simulink model "emerg_imp"  (R2018a)
settings: Solver=FixedStepDiscrete  StartTime=0.0  StopTime=10.0  RelTol=1e-3
settings Model: Creator=BEAR  LastModifiedBy=BEAR
settings OptimizationCC: DefaultParameterBehavior=Inlined  UseDivisionForNetSlopeComputation=on  UseFloatMulNetSlope=on  InlineInvariantSignals=on  PassReuseOutputArgsAs=Individual arguments  ZeroExternalMemoryAtStartup=off  ZeroInternalMemoryAtStartup=off  NoFixptDivByZeroProtection=on  EfficientFloat2IntCast=on  LifeSpan=1  OptimizeBlockOrder=speed  DifferentSizesBufferReuse=on
settings DebuggingCC: ParameterTunabilityLossMsg=error
settings HardwareCC: ProdBitPerLong=64  ProdLongLongMode=on  ProdHWDeviceType=Intel->x86-64 (Mac OS X)
settings SFSimCC: MATLABDynamicMemAlloc=off
settings RTWCC: SystemTargetFile=ert.tlc  TemplateMakefile=ert_default_tmf  GenerateReport=on  IncludeHyperlinkInReport=on  LaunchReport=on  GenerateTraceInfo=on  GenerateTraceReport=on  GenerateTraceReportSl=on  GenerateTraceReportSf=on  GenerateTraceReportEml=on  GenerateCodeMetricsReport=on
settings CodeAppCC: ForceParamTrailComments=on  IgnoreCustomStorageClasses=off  OperatorAnnotations=on  SimulinkDataObjDesc=on  SFDataObjDesc=on  CustomSymbolStrGlobalVar=rt$N$M  CustomSymbolStrType=$N$M  CustomSymbolStrFcn=$N$M$F  CustomSymbolStrMacro=$N$M  InsertBlockDesc=on
settings ERTTargetCC: TargetLangStandard=C99 (ISO)  GenerateSampleERTMain=on  IncludeMdlTerminateFcn=off  CombineSignalStateStructs=on  SupportAbsoluteTime=off  SupportComplex=off  SupportNonInlinedSFcns=on  InlinedParameterPlacement=NonHierarchical  ERTCustomFileTemplate=example_file_process.tlc  ERTFilePackagingFormat=CompactWithDataFile

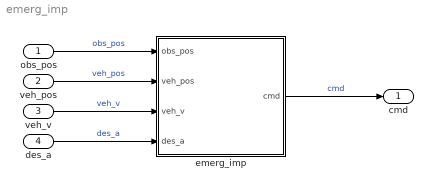
== system emerg_imp ==
  obs_pos : Inport
  veh_pos : Inport  Port=2
  veh_v : Inport  Port=3
  des_a : Inport  Port=4
  emerg_imp : Stateflow chart  TreatAsAtomicUnit=on
  cmd : Outport
  wires:
  obs_pos/1 -> emerg_imp/1(obs_pos)  "obs_pos"
  veh_pos/1 -> emerg_imp/2(veh_pos)  "veh_pos"
  veh_v/1 -> emerg_imp/3(veh_v)  "veh_v"
  des_a/1 -> emerg_imp/4(des_a)  "des_a"
  emerg_imp/1(cmd) -> cmd/1  "cmd"

== stateflow chart emerg_imp/emerg_imp ==
  state state
  (junction 20) -> state [order 2] : /{cmd=min_a}
  (default) -> state
  state -> (junction 14) : {next_v=veh_v+des_a*period;
      |  next_s=veh_pos+veh_v*period
      |               +0.5*des_a*period*period;}
  (junction 14) -> (junction 20) [order 2] : {next_s=veh_pos+veh_v*period}
  (junction 20) -> state [order 1] : [veh_v<=V_lim()]/{cmd=0}
  (junction 14) -> state [order 1] : [next_v<=V_lim()]
      | /{cmd=des_a}
  data: v_lim function_output; max_v constant double =10; min_a constant double =-3; period constant double =0.005; obs_pos input double; veh_pos input double; veh_v input double; des_a input double; cmd output double; next_v local double; next_s local double
  function v_lim = V_lim:
    | function v_lim = V_lim()
    |  
    | distance = obs_pos - next_s;
    | max_d = max_v * max_v / (-2 * min_a);
    | if obs_pos <= 0 || distance >= max_d
    |     v_lim = max_v;
    | else
    |     if distance >= 0
    |         v_lim = sqrt(-2 * min_a * distance);
    |     else
    |         v_lim = 0;
    |     end
    | end
